simulink model "Demo_Intersection_cs"  (Simulink 7.6)
settings: Solver=FixedStepDiscrete  SolverMode=SingleTasking  StartTime=0.0  StopTime=13  FixedStep=1/20  RelTol=1e-3
PreLoadFcn:
  | check_NUTS_defined
  | model_closed = 0;
  | assignin('base',['model_closed_' bdroot],false);
InitFcn:
  | PreScanExperimentInitFcn(bdroot)
StopFcn:
  | PreScanExperimentStopFcn(bdroot);
  | 
undefined symbols (not defined in the file or in its folder): DiscIntNeverNeededParam
libraries: PreScanSimulinkLibrary x32, PreScanUsefulBlocks x8, simulink_extras x3
(part 5 of 5)

== system Demo_Intersection_cs/Nissan_Cabstar_1/Trajectories/Traj2State3/Traj2State2/Traj2MuxState_Ext ==
  Traj : Inport
  Terminator{1..9} (9 alike) : Terminator
  demux : Subsystem
  x [m] : Outport
  y [m] : Outport  Port=2
  z [m] : Outport  Port=3
  dx [m/s] : Outport  Port=4
  dy [m/s] : Outport  Port=5
  dz [m/s] : Outport  Port=6
  R [rad] : Outport  Port=7
  P [rad] : Outport  Port=8
  Y [rad] : Outport  Port=9
  wires:
  demux/9(Y) -> Y [rad]/1
  demux/7(R) -> R [rad]/1
  demux/5(vely) -> dy [m/s]/1
  demux/4(velx) -> dx [m/s]/1
  demux/10(velR) -> Terminator4/1
  demux/11(velP) -> Terminator5/1
  demux/12(velY) -> Terminator1/1
  demux/13(accx) -> Terminator8/1
  demux/14(accy) -> Terminator9/1
  demux/15(accz) -> Terminator7/1
  demux/18(accY) -> Terminator2/1
  demux/16(accR) -> Terminator3/1
  demux/17(accP) -> Terminator6/1
  demux/3(z) -> z [m]/1
  Traj/1 -> demux/1(traj)
  demux/6(velz) -> dz [m/s]/1
  demux/1(x) -> x [m]/1
  demux/2(y) -> y [m]/1
  demux/8(P) -> P [rad]/1

== system Demo_Intersection_cs/Toyota_Previa_1/Trajectories/Traj2State1/Traj2State2/MuxState ==
  x [m] : Inport
  y [m] : Inport  Port=2
  z [m] : Inport  Port=3
  dx [m/s] : Inport  Port=4
  dy [m/s] : Inport  Port=5
  dz [m/s] : Inport  Port=6
  R [rad] : Inport  Port=7
  P [rad] : Inport  Port=8
  Y [rad] : Inport  Port=9
  Mux : Mux  Inputs=9
  state : Outport
  wires:
  z [m]/1 -> Mux/3
  y [m]/1 -> Mux/2
  x [m]/1 -> Mux/1
  Y [rad]/1 -> Mux/9
  P [rad]/1 -> Mux/8
  R [rad]/1 -> Mux/7
  dz [m/s]/1 -> Mux/6
  dy [m/s]/1 -> Mux/5
  dx [m/s]/1 -> Mux/4
  Mux/1 -> state/1

== system Demo_Intersection_cs/Toyota_Previa_1/Trajectories/Traj2State1/Traj2State2/Traj2MuxState_Ext ==
  Traj : Inport
  Terminator{1..9} (9 alike) : Terminator
  demux : Subsystem
  x [m] : Outport
  y [m] : Outport  Port=2
  z [m] : Outport  Port=3
  dx [m/s] : Outport  Port=4
  dy [m/s] : Outport  Port=5
  dz [m/s] : Outport  Port=6
  R [rad] : Outport  Port=7
  P [rad] : Outport  Port=8
  Y [rad] : Outport  Port=9
  wires:
  demux/9(Y) -> Y [rad]/1
  demux/7(R) -> R [rad]/1
  demux/5(vely) -> dy [m/s]/1
  demux/4(velx) -> dx [m/s]/1
  demux/10(velR) -> Terminator4/1
  demux/11(velP) -> Terminator5/1
  demux/12(velY) -> Terminator1/1
  demux/13(accx) -> Terminator8/1
  demux/14(accy) -> Terminator9/1
  demux/15(accz) -> Terminator7/1
  demux/18(accY) -> Terminator2/1
  demux/16(accR) -> Terminator3/1
  demux/17(accP) -> Terminator6/1
  demux/3(z) -> z [m]/1
  Traj/1 -> demux/1(traj)
  demux/6(velz) -> dz [m/s]/1
  demux/1(x) -> x [m]/1
  demux/2(y) -> y [m]/1
  demux/8(P) -> P [rad]/1

== system Demo_Intersection_cs/Toyota_Previa_1/Trajectories/Traj2State2/Traj2State2/MuxState ==
  x [m] : Inport
  y [m] : Inport  Port=2
  z [m] : Inport  Port=3
  dx [m/s] : Inport  Port=4
  dy [m/s] : Inport  Port=5
  dz [m/s] : Inport  Port=6
  R [rad] : Inport  Port=7
  P [rad] : Inport  Port=8
  Y [rad] : Inport  Port=9
  Mux : Mux  Inputs=9
  state : Outport
  wires:
  z [m]/1 -> Mux/3
  y [m]/1 -> Mux/2
  x [m]/1 -> Mux/1
  Y [rad]/1 -> Mux/9
  P [rad]/1 -> Mux/8
  R [rad]/1 -> Mux/7
  dz [m/s]/1 -> Mux/6
  dy [m/s]/1 -> Mux/5
  dx [m/s]/1 -> Mux/4
  Mux/1 -> state/1

== system Demo_Intersection_cs/Toyota_Previa_1/Trajectories/Traj2State2/Traj2State2/Traj2MuxState_Ext ==
  Traj : Inport
  Terminator{1..9} (9 alike) : Terminator
  demux : Subsystem
  x [m] : Outport
  y [m] : Outport  Port=2
  z [m] : Outport  Port=3
  dx [m/s] : Outport  Port=4
  dy [m/s] : Outport  Port=5
  dz [m/s] : Outport  Port=6
  R [rad] : Outport  Port=7
  P [rad] : Outport  Port=8
  Y [rad] : Outport  Port=9
  wires:
  demux/9(Y) -> Y [rad]/1
  demux/7(R) -> R [rad]/1
  demux/5(vely) -> dy [m/s]/1
  demux/4(velx) -> dx [m/s]/1
  demux/10(velR) -> Terminator4/1
  demux/11(velP) -> Terminator5/1
  demux/12(velY) -> Terminator1/1
  demux/13(accx) -> Terminator8/1
  demux/14(accy) -> Terminator9/1
  demux/15(accz) -> Terminator7/1
  demux/18(accY) -> Terminator2/1
  demux/16(accR) -> Terminator3/1
  demux/17(accP) -> Terminator6/1
  demux/3(z) -> z [m]/1
  Traj/1 -> demux/1(traj)
  demux/6(velz) -> dz [m/s]/1
  demux/1(x) -> x [m]/1
  demux/2(y) -> y [m]/1
  demux/8(P) -> P [rad]/1

== system Demo_Intersection_cs/Toyota_Previa_1/Trajectories/Traj2State3/Traj2State2/MuxState ==
  x [m] : Inport
  y [m] : Inport  Port=2
  z [m] : Inport  Port=3
  dx [m/s] : Inport  Port=4
  dy [m/s] : Inport  Port=5
  dz [m/s] : Inport  Port=6
  R [rad] : Inport  Port=7
  P [rad] : Inport  Port=8
  Y [rad] : Inport  Port=9
  Mux : Mux  Inputs=9
  state : Outport
  wires:
  z [m]/1 -> Mux/3
  y [m]/1 -> Mux/2
  x [m]/1 -> Mux/1
  Y [rad]/1 -> Mux/9
  P [rad]/1 -> Mux/8
  R [rad]/1 -> Mux/7
  dz [m/s]/1 -> Mux/6
  dy [m/s]/1 -> Mux/5
  dx [m/s]/1 -> Mux/4
  Mux/1 -> state/1

== system Demo_Intersection_cs/Toyota_Previa_1/Trajectories/Traj2State3/Traj2State2/Traj2MuxState_Ext ==
  Traj : Inport
  Terminator{1..9} (9 alike) : Terminator
  demux : Subsystem
  x [m] : Outport
  y [m] : Outport  Port=2
  z [m] : Outport  Port=3
  dx [m/s] : Outport  Port=4
  dy [m/s] : Outport  Port=5
  dz [m/s] : Outport  Port=6
  R [rad] : Outport  Port=7
  P [rad] : Outport  Port=8
  Y [rad] : Outport  Port=9
  wires:
  demux/9(Y) -> Y [rad]/1
  demux/7(R) -> R [rad]/1
  demux/5(vely) -> dy [m/s]/1
  demux/4(velx) -> dx [m/s]/1
  demux/10(velR) -> Terminator4/1
  demux/11(velP) -> Terminator5/1
  demux/12(velY) -> Terminator1/1
  demux/13(accx) -> Terminator8/1
  demux/14(accy) -> Terminator9/1
  demux/15(accz) -> Terminator7/1
  demux/18(accY) -> Terminator2/1
  demux/16(accR) -> Terminator3/1
  demux/17(accP) -> Terminator6/1
  demux/3(z) -> z [m]/1
  Traj/1 -> demux/1(traj)
  demux/6(velz) -> dz [m/s]/1
  demux/1(x) -> x [m]/1
  demux/2(y) -> y [m]/1
  demux/8(P) -> P [rad]/1

== system Demo_Intersection_cs/Toyota_Yaris_1/Trajectories/Traj2State1/Traj2State2/MuxState ==
  x [m] : Inport
  y [m] : Inport  Port=2
  z [m] : Inport  Port=3
  dx [m/s] : Inport  Port=4
  dy [m/s] : Inport  Port=5
  dz [m/s] : Inport  Port=6
  R [rad] : Inport  Port=7
  P [rad] : Inport  Port=8
  Y [rad] : Inport  Port=9
  Mux : Mux  Inputs=9
  state : Outport
  wires:
  z [m]/1 -> Mux/3
  y [m]/1 -> Mux/2
  x [m]/1 -> Mux/1
  Y [rad]/1 -> Mux/9
  P [rad]/1 -> Mux/8
  R [rad]/1 -> Mux/7
  dz [m/s]/1 -> Mux/6
  dy [m/s]/1 -> Mux/5
  dx [m/s]/1 -> Mux/4
  Mux/1 -> state/1

== system Demo_Intersection_cs/Toyota_Yaris_1/Trajectories/Traj2State1/Traj2State2/Traj2MuxState_Ext ==
  Traj : Inport
  Terminator{1..9} (9 alike) : Terminator
  demux : Subsystem
  x [m] : Outport
  y [m] : Outport  Port=2
  z [m] : Outport  Port=3
  dx [m/s] : Outport  Port=4
  dy [m/s] : Outport  Port=5
  dz [m/s] : Outport  Port=6
  R [rad] : Outport  Port=7
  P [rad] : Outport  Port=8
  Y [rad] : Outport  Port=9
  wires:
  demux/9(Y) -> Y [rad]/1
  demux/7(R) -> R [rad]/1
  demux/5(vely) -> dy [m/s]/1
  demux/4(velx) -> dx [m/s]/1
  demux/10(velR) -> Terminator4/1
  demux/11(velP) -> Terminator5/1
  demux/12(velY) -> Terminator1/1
  demux/13(accx) -> Terminator8/1
  demux/14(accy) -> Terminator9/1
  demux/15(accz) -> Terminator7/1
  demux/18(accY) -> Terminator2/1
  demux/16(accR) -> Terminator3/1
  demux/17(accP) -> Terminator6/1
  demux/3(z) -> z [m]/1
  Traj/1 -> demux/1(traj)
  demux/6(velz) -> dz [m/s]/1
  demux/1(x) -> x [m]/1
  demux/2(y) -> y [m]/1
  demux/8(P) -> P [rad]/1

== system Demo_Intersection_cs/Toyota_Yaris_1/Trajectories/Traj2State2/Traj2State2/MuxState ==
  x [m] : Inport
  y [m] : Inport  Port=2
  z [m] : Inport  Port=3
  dx [m/s] : Inport  Port=4
  dy [m/s] : Inport  Port=5
  dz [m/s] : Inport  Port=6
  R [rad] : Inport  Port=7
  P [rad] : Inport  Port=8
  Y [rad] : Inport  Port=9
  Mux : Mux  Inputs=9
  state : Outport
  wires:
  z [m]/1 -> Mux/3
  y [m]/1 -> Mux/2
  x [m]/1 -> Mux/1
  Y [rad]/1 -> Mux/9
  P [rad]/1 -> Mux/8
  R [rad]/1 -> Mux/7
  dz [m/s]/1 -> Mux/6
  dy [m/s]/1 -> Mux/5
  dx [m/s]/1 -> Mux/4
  Mux/1 -> state/1

== system Demo_Intersection_cs/Toyota_Yaris_1/Trajectories/Traj2State2/Traj2State2/Traj2MuxState_Ext ==
  Traj : Inport
  Terminator{1..9} (9 alike) : Terminator
  demux : Subsystem
  x [m] : Outport
  y [m] : Outport  Port=2
  z [m] : Outport  Port=3
  dx [m/s] : Outport  Port=4
  dy [m/s] : Outport  Port=5
  dz [m/s] : Outport  Port=6
  R [rad] : Outport  Port=7
  P [rad] : Outport  Port=8
  Y [rad] : Outport  Port=9
  wires:
  demux/9(Y) -> Y [rad]/1
  demux/7(R) -> R [rad]/1
  demux/5(vely) -> dy [m/s]/1
  demux/4(velx) -> dx [m/s]/1
  demux/10(velR) -> Terminator4/1
  demux/11(velP) -> Terminator5/1
  demux/12(velY) -> Terminator1/1
  demux/13(accx) -> Terminator8/1
  demux/14(accy) -> Terminator9/1
  demux/15(accz) -> Terminator7/1
  demux/18(accY) -> Terminator2/1
  demux/16(accR) -> Terminator3/1
  demux/17(accP) -> Terminator6/1
  demux/3(z) -> z [m]/1
  Traj/1 -> demux/1(traj)
  demux/6(velz) -> dz [m/s]/1
  demux/1(x) -> x [m]/1
  demux/2(y) -> y [m]/1
  demux/8(P) -> P [rad]/1

== system Demo_Intersection_cs/Toyota_Yaris_1/Trajectories/Traj2State3/Traj2State2/MuxState ==
  x [m] : Inport
  y [m] : Inport  Port=2
  z [m] : Inport  Port=3
  dx [m/s] : Inport  Port=4
  dy [m/s] : Inport  Port=5
  dz [m/s] : Inport  Port=6
  R [rad] : Inport  Port=7
  P [rad] : Inport  Port=8
  Y [rad] : Inport  Port=9
  Mux : Mux  Inputs=9
  state : Outport
  wires:
  z [m]/1 -> Mux/3
  y [m]/1 -> Mux/2
  x [m]/1 -> Mux/1
  Y [rad]/1 -> Mux/9
  P [rad]/1 -> Mux/8
  R [rad]/1 -> Mux/7
  dz [m/s]/1 -> Mux/6
  dy [m/s]/1 -> Mux/5
  dx [m/s]/1 -> Mux/4
  Mux/1 -> state/1

== system Demo_Intersection_cs/Toyota_Yaris_1/Trajectories/Traj2State3/Traj2State2/Traj2MuxState_Ext ==
  Traj : Inport
  Terminator{1..9} (9 alike) : Terminator
  demux : Subsystem
  x [m] : Outport
  y [m] : Outport  Port=2
  z [m] : Outport  Port=3
  dx [m/s] : Outport  Port=4
  dy [m/s] : Outport  Port=5
  dz [m/s] : Outport  Port=6
  R [rad] : Outport  Port=7
  P [rad] : Outport  Port=8
  Y [rad] : Outport  Port=9
  wires:
  demux/9(Y) -> Y [rad]/1
  demux/7(R) -> R [rad]/1
  demux/5(vely) -> dy [m/s]/1
  demux/4(velx) -> dx [m/s]/1
  demux/10(velR) -> Terminator4/1
  demux/11(velP) -> Terminator5/1
  demux/12(velY) -> Terminator1/1
  demux/13(accx) -> Terminator8/1
  demux/14(accy) -> Terminator9/1
  demux/15(accz) -> Terminator7/1
  demux/18(accY) -> Terminator2/1
  demux/16(accR) -> Terminator3/1
  demux/17(accP) -> Terminator6/1
  demux/3(z) -> z [m]/1
  Traj/1 -> demux/1(traj)
  demux/6(velz) -> dz [m/s]/1
  demux/1(x) -> x [m]/1
  demux/2(y) -> y [m]/1
  demux/8(P) -> P [rad]/1

== system Demo_Intersection_cs/Nissan_Cabstar_1/Trajectories/Traj2State1/Traj2State2/Traj2MuxState_Ext/demux ==
  traj : Inport
  Demux : Demux  Outputs=18
  x : Outport
  y : Outport  Port=2
  z : Outport  Port=3
  velx : Outport  Port=4
  vely : Outport  Port=5
  velz : Outport  Port=6
  R : Outport  Port=7
  P : Outport  Port=8
  Y : Outport  Port=9
  velR : Outport  Port=10
  velP : Outport  Port=11
  velY : Outport  Port=12
  accx : Outport  Port=13
  accy : Outport  Port=14
  accz : Outport  Port=15
  accR : Outport  Port=16
  accP : Outport  Port=17
  accY : Outport  Port=18
  wires:
  Demux/18 -> accY/1
  Demux/17 -> accP/1
  Demux/16 -> accR/1
  Demux/15 -> accz/1
  Demux/14 -> accy/1
  Demux/13 -> accx/1
  Demux/12 -> velY/1
  Demux/11 -> velP/1
  Demux/10 -> velR/1
  Demux/9 -> velz/1
  Demux/8 -> vely/1
  Demux/7 -> velx/1
  Demux/6 -> Y/1
  Demux/5 -> P/1
  traj/1 -> Demux/1
  Demux/4 -> R/1
  Demux/3 -> z/1
  Demux/2 -> y/1
  Demux/1 -> x/1

== system Demo_Intersection_cs/Nissan_Cabstar_1/Trajectories/Traj2State2/Traj2State2/Traj2MuxState_Ext/demux ==
  traj : Inport
  Demux : Demux  Outputs=18
  x : Outport
  y : Outport  Port=2
  z : Outport  Port=3
  velx : Outport  Port=4
  vely : Outport  Port=5
  velz : Outport  Port=6
  R : Outport  Port=7
  P : Outport  Port=8
  Y : Outport  Port=9
  velR : Outport  Port=10
  velP : Outport  Port=11
  velY : Outport  Port=12
  accx : Outport  Port=13
  accy : Outport  Port=14
  accz : Outport  Port=15
  accR : Outport  Port=16
  accP : Outport  Port=17
  accY : Outport  Port=18
  wires:
  Demux/18 -> accY/1
  Demux/17 -> accP/1
  Demux/16 -> accR/1
  Demux/15 -> accz/1
  Demux/14 -> accy/1
  Demux/13 -> accx/1
  Demux/12 -> velY/1
  Demux/11 -> velP/1
  Demux/10 -> velR/1
  Demux/9 -> velz/1
  Demux/8 -> vely/1
  Demux/7 -> velx/1
  Demux/6 -> Y/1
  Demux/5 -> P/1
  traj/1 -> Demux/1
  Demux/4 -> R/1
  Demux/3 -> z/1
  Demux/2 -> y/1
  Demux/1 -> x/1

== system Demo_Intersection_cs/Nissan_Cabstar_1/Trajectories/Traj2State3/Traj2State2/Traj2MuxState_Ext/demux ==
  traj : Inport
  Demux : Demux  Outputs=18
  x : Outport
  y : Outport  Port=2
  z : Outport  Port=3
  velx : Outport  Port=4
  vely : Outport  Port=5
  velz : Outport  Port=6
  R : Outport  Port=7
  P : Outport  Port=8
  Y : Outport  Port=9
  velR : Outport  Port=10
  velP : Outport  Port=11
  velY : Outport  Port=12
  accx : Outport  Port=13
  accy : Outport  Port=14
  accz : Outport  Port=15
  accR : Outport  Port=16
  accP : Outport  Port=17
  accY : Outport  Port=18
  wires:
  Demux/18 -> accY/1
  Demux/17 -> accP/1
  Demux/16 -> accR/1
  Demux/15 -> accz/1
  Demux/14 -> accy/1
  Demux/13 -> accx/1
  Demux/12 -> velY/1
  Demux/11 -> velP/1
  Demux/10 -> velR/1
  Demux/9 -> velz/1
  Demux/8 -> vely/1
  Demux/7 -> velx/1
  Demux/6 -> Y/1
  Demux/5 -> P/1
  traj/1 -> Demux/1
  Demux/4 -> R/1
  Demux/3 -> z/1
  Demux/2 -> y/1
  Demux/1 -> x/1

== system Demo_Intersection_cs/Toyota_Previa_1/Trajectories/Traj2State1/Traj2State2/Traj2MuxState_Ext/demux ==
  traj : Inport
  Demux : Demux  Outputs=18
  x : Outport
  y : Outport  Port=2
  z : Outport  Port=3
  velx : Outport  Port=4
  vely : Outport  Port=5
  velz : Outport  Port=6
  R : Outport  Port=7
  P : Outport  Port=8
  Y : Outport  Port=9
  velR : Outport  Port=10
  velP : Outport  Port=11
  velY : Outport  Port=12
  accx : Outport  Port=13
  accy : Outport  Port=14
  accz : Outport  Port=15
  accR : Outport  Port=16
  accP : Outport  Port=17
  accY : Outport  Port=18
  wires:
  Demux/18 -> accY/1
  Demux/17 -> accP/1
  Demux/16 -> accR/1
  Demux/15 -> accz/1
  Demux/14 -> accy/1
  Demux/13 -> accx/1
  Demux/12 -> velY/1
  Demux/11 -> velP/1
  Demux/10 -> velR/1
  Demux/9 -> velz/1
  Demux/8 -> vely/1
  Demux/7 -> velx/1
  Demux/6 -> Y/1
  Demux/5 -> P/1
  traj/1 -> Demux/1
  Demux/4 -> R/1
  Demux/3 -> z/1
  Demux/2 -> y/1
  Demux/1 -> x/1

== system Demo_Intersection_cs/Toyota_Previa_1/Trajectories/Traj2State2/Traj2State2/Traj2MuxState_Ext/demux ==
  traj : Inport
  Demux : Demux  Outputs=18
  x : Outport
  y : Outport  Port=2
  z : Outport  Port=3
  velx : Outport  Port=4
  vely : Outport  Port=5
  velz : Outport  Port=6
  R : Outport  Port=7
  P : Outport  Port=8
  Y : Outport  Port=9
  velR : Outport  Port=10
  velP : Outport  Port=11
  velY : Outport  Port=12
  accx : Outport  Port=13
  accy : Outport  Port=14
  accz : Outport  Port=15
  accR : Outport  Port=16
  accP : Outport  Port=17
  accY : Outport  Port=18
  wires:
  Demux/18 -> accY/1
  Demux/17 -> accP/1
  Demux/16 -> accR/1
  Demux/15 -> accz/1
  Demux/14 -> accy/1
  Demux/13 -> accx/1
  Demux/12 -> velY/1
  Demux/11 -> velP/1
  Demux/10 -> velR/1
  Demux/9 -> velz/1
  Demux/8 -> vely/1
  Demux/7 -> velx/1
  Demux/6 -> Y/1
  Demux/5 -> P/1
  traj/1 -> Demux/1
  Demux/4 -> R/1
  Demux/3 -> z/1
  Demux/2 -> y/1
  Demux/1 -> x/1

== system Demo_Intersection_cs/Toyota_Previa_1/Trajectories/Traj2State3/Traj2State2/Traj2MuxState_Ext/demux ==
  traj : Inport
  Demux : Demux  Outputs=18
  x : Outport
  y : Outport  Port=2
  z : Outport  Port=3
  velx : Outport  Port=4
  vely : Outport  Port=5
  velz : Outport  Port=6
  R : Outport  Port=7
  P : Outport  Port=8
  Y : Outport  Port=9
  velR : Outport  Port=10
  velP : Outport  Port=11
  velY : Outport  Port=12
  accx : Outport  Port=13
  accy : Outport  Port=14
  accz : Outport  Port=15
  accR : Outport  Port=16
  accP : Outport  Port=17
  accY : Outport  Port=18
  wires:
  Demux/18 -> accY/1
  Demux/17 -> accP/1
  Demux/16 -> accR/1
  Demux/15 -> accz/1
  Demux/14 -> accy/1
  Demux/13 -> accx/1
  Demux/12 -> velY/1
  Demux/11 -> velP/1
  Demux/10 -> velR/1
  Demux/9 -> velz/1
  Demux/8 -> vely/1
  Demux/7 -> velx/1
  Demux/6 -> Y/1
  Demux/5 -> P/1
  traj/1 -> Demux/1
  Demux/4 -> R/1
  Demux/3 -> z/1
  Demux/2 -> y/1
  Demux/1 -> x/1

== system Demo_Intersection_cs/Toyota_Yaris_1/Trajectories/Traj2State1/Traj2State2/Traj2MuxState_Ext/demux ==
  traj : Inport
  Demux : Demux  Outputs=18
  x : Outport
  y : Outport  Port=2
  z : Outport  Port=3
  velx : Outport  Port=4
  vely : Outport  Port=5
  velz : Outport  Port=6
  R : Outport  Port=7
  P : Outport  Port=8
  Y : Outport  Port=9
  velR : Outport  Port=10
  velP : Outport  Port=11
  velY : Outport  Port=12
  accx : Outport  Port=13
  accy : Outport  Port=14
  accz : Outport  Port=15
  accR : Outport  Port=16
  accP : Outport  Port=17
  accY : Outport  Port=18
  wires:
  Demux/18 -> accY/1
  Demux/17 -> accP/1
  Demux/16 -> accR/1
  Demux/15 -> accz/1
  Demux/14 -> accy/1
  Demux/13 -> accx/1
  Demux/12 -> velY/1
  Demux/11 -> velP/1
  Demux/10 -> velR/1
  Demux/9 -> velz/1
  Demux/8 -> vely/1
  Demux/7 -> velx/1
  Demux/6 -> Y/1
  Demux/5 -> P/1
  traj/1 -> Demux/1
  Demux/4 -> R/1
  Demux/3 -> z/1
  Demux/2 -> y/1
  Demux/1 -> x/1

== system Demo_Intersection_cs/Toyota_Yaris_1/Trajectories/Traj2State2/Traj2State2/Traj2MuxState_Ext/demux ==
  traj : Inport
  Demux : Demux  Outputs=18
  x : Outport
  y : Outport  Port=2
  z : Outport  Port=3
  velx : Outport  Port=4
  vely : Outport  Port=5
  velz : Outport  Port=6
  R : Outport  Port=7
  P : Outport  Port=8
  Y : Outport  Port=9
  velR : Outport  Port=10
  velP : Outport  Port=11
  velY : Outport  Port=12
  accx : Outport  Port=13
  accy : Outport  Port=14
  accz : Outport  Port=15
  accR : Outport  Port=16
  accP : Outport  Port=17
  accY : Outport  Port=18
  wires:
  Demux/18 -> accY/1
  Demux/17 -> accP/1
  Demux/16 -> accR/1
  Demux/15 -> accz/1
  Demux/14 -> accy/1
  Demux/13 -> accx/1
  Demux/12 -> velY/1
  Demux/11 -> velP/1
  Demux/10 -> velR/1
  Demux/9 -> velz/1
  Demux/8 -> vely/1
  Demux/7 -> velx/1
  Demux/6 -> Y/1
  Demux/5 -> P/1
  traj/1 -> Demux/1
  Demux/4 -> R/1
  Demux/3 -> z/1
  Demux/2 -> y/1
  Demux/1 -> x/1

== system Demo_Intersection_cs/Toyota_Yaris_1/Trajectories/Traj2State3/Traj2State2/Traj2MuxState_Ext/demux ==
  traj : Inport
  Demux : Demux  Outputs=18
  x : Outport
  y : Outport  Port=2
  z : Outport  Port=3
  velx : Outport  Port=4
  vely : Outport  Port=5
  velz : Outport  Port=6
  R : Outport  Port=7
  P : Outport  Port=8
  Y : Outport  Port=9
  velR : Outport  Port=10
  velP : Outport  Port=11
  velY : Outport  Port=12
  accx : Outport  Port=13
  accy : Outport  Port=14
  accz : Outport  Port=15
  accR : Outport  Port=16
  accP : Outport  Port=17
  accY : Outport  Port=18
  wires:
  Demux/18 -> accY/1
  Demux/17 -> accP/1
  Demux/16 -> accR/1
  Demux/15 -> accz/1
  Demux/14 -> accy/1
  Demux/13 -> accx/1
  Demux/12 -> velY/1
  Demux/11 -> velP/1
  Demux/10 -> velR/1
  Demux/9 -> velz/1
  Demux/8 -> vely/1
  Demux/7 -> velx/1
  Demux/6 -> Y/1
  Demux/5 -> P/1
  traj/1 -> Demux/1
  Demux/4 -> R/1
  Demux/3 -> z/1
  Demux/2 -> y/1
  Demux/1 -> x/1

== matlab function Mazda_RX8_1/Sort AIR Output based on ID/Embedded MATLAB Function ==
  data: u input double; y output double; mode input double; ignorezero input double; ids input double
function y = fcn(u,mode, ignorezero, ids)
% This block supports an embeddable subset of the MATLAB language.
% See the help menu for details. 

[a,y] = sort(u);
if mode == 2 %'descend'
    y=y(end:-1:1);
end

if mode == 1 && ignorezero == 1 
    ly = length(y);
    % ignore zero detections (NB: not required for descending)
    % => place zero detections at end
% TODO: preferred implementation: not available yet in 2006a
%     A=logical(ids(y)~=0);
%     y=[y(A); y(~A)]';
    index=ly+1;
    base=0; %temp value to fix issue with loop variable i
    indices = zeros(1,ly);
    for i=1:ly
        base=i;
        if ids(y(i)) ~= 0
            index = i;
            break
        end
    end
    for i=1:ly-index+1
        indices(i) = index+i-1;
    end
    if index==ly+1;
        base=0;
    end
    for j=1:index-1
        indices(base+j)=j;
    end
    y=y(indices);
end

== stateflow chart Mazda_RX8_1/Decision Algorithm ==
  state Decision_algorithm
    state CAR1 [parallel]
      settings: executionOrder=2
      state Lane1
        state RightTurn
          en: W[1]=WM[1];
        state Straight
          en: W[1]=WM[2];
        state LeftTurn
          en: W[1]=WM[3];
        (default) -> (junction 56) [order 1]
        (junction 56) -> Decision_algorithm.CAR1.Lane1.Straight [order 2] : [C1[3]==0]
        (junction 56) -> Decision_algorithm.CAR1.Lane1.LeftTurn [order 1] : [C1[3]<0]
        (junction 56) -> Decision_algorithm.CAR1.Lane1.RightTurn [order 3] : [C1[3]>0]
        (default) -> Decision_algorithm.CAR1.Lane1.Straight [order 2]
      state Lane2
        state LeftTurn
          en: W[2]=WM[6];
        state Straight
          en: W[2]=WM[5];
        state RightTurn
          en: W[2]=WM[4];
        (default) -> (junction 57) [order 1]
        (junction 57) -> Decision_algorithm.CAR1.Lane2.RightTurn [order 3] : [C1[3]>0]
        (junction 57) -> Decision_algorithm.CAR1.Lane2.LeftTurn [order 1] : [C1[3]<0]
        (junction 57) -> Decision_algorithm.CAR1.Lane2.Straight [order 2] : [C1[3]==0]
        (default) -> Decision_algorithm.CAR1.Lane2.Straight [order 2]
      state Enter
      state Lane3
        state RightTurn
          en: W[3]=WM[7];
        state Straight
          en: W[3]=WM[8];
        state LeftTurn
          en: W[3]=WM[9];
        (junction 58) -> Decision_algorithm.CAR1.Lane3.RightTurn [order 1] : [C1[3]>0]
        (junction 58) -> Decision_algorithm.CAR1.Lane3.Straight [order 3] : [C1[3]==0]
        (junction 58) -> Decision_algorithm.CAR1.Lane3.LeftTurn [order 2] : [C1[3]<0]
        (default) -> (junction 58) [order 1]
        (default) -> Decision_algorithm.CAR1.Lane3.Straight [order 2]
      Decision_algorithm.CAR1.Enter -> Decision_algorithm.CAR1.Lane3 [order 2] : [C1[2]>-135 && C1[2]<-90 && C1[1]<Rcross...
          | && ((C1[4]>315 && C1[4]<=360) ||...
          | (C1[4]>=0 && C1[4]<45))]
      Decision_algorithm.CAR1.Enter -> Decision_algorithm.CAR1.Lane1 [order 3] : [C1[2]>45 && C1[2]<90 && C1[1]<Rcross...
          | && C1[4]>135 && C1[4]<225]
      Decision_algorithm.CAR1.Enter -> Decision_algorithm.CAR1.Lane2 [order 1] : [C1[2]>-45 && C1[2]<0 && C1[1]<Rcross...
          | && C1[4]>225 && C1[4]<315]
      (default) -> Decision_algorithm.CAR1.Enter : {W[1]=0;
          | W[2]=0;
          | W[3]=0;}
      Decision_algorithm.CAR1.Lane3.Straight -> Decision_algorithm.CAR1.Enter
      Decision_algorithm.CAR1.Lane3.RightTurn -> Decision_algorithm.CAR1.Enter
      Decision_algorithm.CAR1.Lane2.RightTurn -> Decision_algorithm.CAR1.Enter
      Decision_algorithm.CAR1.Lane1.RightTurn -> Decision_algorithm.CAR1.Enter
      Decision_algorithm.CAR1.Lane2.LeftTurn -> Decision_algorithm.CAR1.Enter
      Decision_algorithm.CAR1.Lane2.Straight -> Decision_algorithm.CAR1.Enter
      Decision_algorithm.CAR1.Lane1.Straight -> Decision_algorithm.CAR1.Enter
      Decision_algorithm.CAR1.Lane1.LeftTurn -> Decision_algorithm.CAR1.Enter
      Decision_algorithm.CAR1.Lane3.LeftTurn -> Decision_algorithm.CAR1.Enter
      Decision_algorithm.CAR1.Enter -> Decision_algorithm.CAR1.Enter [order 4] : {W[1]=0;
          | W[2]=0;
          | W[3]=0;}
    state CAR2 [parallel]
      settings: executionOrder=1
      state Lane2
        state LeftTurn
          en: W[5]=WM[6];
        state Straight
          en: W[5]=WM[5];
        state RightTurn
          en: W[5]=WM[4];
        (junction 60) -> Decision_algorithm.CAR2.Lane2.Straight [order 2] : [C2[3]==0]
        (junction 60) -> Decision_algorithm.CAR2.Lane2.LeftTurn [order 1] : [C2[3]<0]
        (junction 60) -> Decision_algorithm.CAR2.Lane2.RightTurn [order 3] : [C2[3]>0]
        (default) -> (junction 60) [order 1]
        (default) -> Decision_algorithm.CAR2.Lane2.Straight [order 2]
      state Lane1
        state RightTurn
          en: W[4]=WM[1];
        state Straight
          en: W[4]=WM[2];
        state LeftTurn
          en: W[4]=WM[3];
        (junction 61) -> Decision_algorithm.CAR2.Lane1.RightTurn [order 2] : [C2[3]>0]
        (junction 61) -> Decision_algorithm.CAR2.Lane1.LeftTurn [order 3] : [C2[3]<0]
        (junction 61) -> Decision_algorithm.CAR2.Lane1.Straight [order 1] : [C2[3]==0]
        (default) -> (junction 61) [order 1]
        (default) -> Decision_algorithm.CAR2.Lane1.Straight [order 2]
      state Lane3
        state LeftTurn
          en: W[6]=WM[9];
        state Straight
          en: W[6]=WM[8];
        state RightTurn
          en: W[6]=WM[7];
        (default) -> (junction 59) [order 1]
        (junction 59) -> Decision_algorithm.CAR2.Lane3.LeftTurn [order 2] : [C2[3]<0]
        (junction 59) -> Decision_algorithm.CAR2.Lane3.Straight [order 3] : [C2[3]==0]
        (junction 59) -> Decision_algorithm.CAR2.Lane3.RightTurn [order 1] : [C2[3]>0]
        (default) -> Decision_algorithm.CAR2.Lane3.Straight [order 2]
      state Enter
      Decision_algorithm.CAR2.Lane3.Straight -> Decision_algorithm.CAR2.Enter
      (default) -> Decision_algorithm.CAR2.Enter : {W[4]=0;
          | W[5]=0;
          | W[6]=0;}
      Decision_algorithm.CAR2.Enter -> Decision_algorithm.CAR2.Lane2 [order 1] : [C2[2]>-45 && C2[2]<0 && C2[1]<Rcross...
          | && C2[4]>225 && C2[4]<315]
      Decision_algorithm.CAR2.Enter -> Decision_algorithm.CAR2.Lane1 [order 3] : [C2[2]>45 && C2[2]<90 && C2[1]<Rcross...
          | && C2[4]>135 && C2[4]<225]
      Decision_algorithm.CAR2.Enter -> Decision_algorithm.CAR2.Lane3 [order 2] : [C2[2]>-135 && C2[2]<-90 && C2[1]<Rcross...
          | && ((C2[4]>315 && C2[4]<=360) ||...
          | (C2[4]>=0 && C2[4]<45))]
      Decision_algorithm.CAR2.Lane2.RightTurn -> Decision_algorithm.CAR2.Enter
      Decision_algorithm.CAR2.Lane1.RightTurn -> Decision_algorithm.CAR2.Enter
      Decision_algorithm.CAR2.Lane3.RightTurn -> Decision_algorithm.CAR2.Enter
      Decision_algorithm.CAR2.Lane3.LeftTurn -> Decision_algorithm.CAR2.Enter
      Decision_algorithm.CAR2.Lane1.LeftTurn -> Decision_algorithm.CAR2.Enter
      Decision_algorithm.CAR2.Lane1.Straight -> Decision_algorithm.CAR2.Enter
      Decision_algorithm.CAR2.Lane2.Straight -> Decision_algorithm.CAR2.Enter
      Decision_algorithm.CAR2.Lane2.LeftTurn -> Decision_algorithm.CAR2.Enter
      Decision_algorithm.CAR2.Enter -> Decision_algorithm.CAR2.Enter [order 4] : {W[4]=0;
          | W[5]=0;
          | W[6]=0;}
    state CAR3 [parallel]
      settings: executionOrder=3
      state Enter
      state Lane3
        state LeftTurn
          en: W[9]=WM[9];
        state Straight
          en: W[9]=WM[8];
        state RightTurn
          en: W[9]=WM[7];
        (default) -> (junction 63) [order 1]
        (junction 63) -> Decision_algorithm.CAR3.Lane3.Straight [order 3] : [C3[3]==0]
        (junction 63) -> Decision_algorithm.CAR3.Lane3.LeftTurn [order 2] : [C3[3]<0]
        (junction 63) -> Decision_algorithm.CAR3.Lane3.RightTurn [order 1] : [C3[3]>0]
        (default) -> Decision_algorithm.CAR3.Lane3.Straight [order 2]
      state Lane2
        state LeftTurn
          en: W[8]=WM[6];
        state Straight
          en: W[8]=WM[5];
        state RightTurn
          en: W[8]=WM[4];
        (junction 64) -> Decision_algorithm.CAR3.Lane2.RightTurn [order 3] : [C3[3]>0]
        (junction 64) -> Decision_algorithm.CAR3.Lane2.Straight [order 2] : [C3[3]==0]
        (junction 64) -> Decision_algorithm.CAR3.Lane2.LeftTurn [order 1] : [C3[3]<0]
        (default) -> (junction 64) [order 1]
        (default) -> Decision_algorithm.CAR3.Lane2.Straight [order 2]
      state Lane1
        state RightTurn
          en: W[7]=WM[1];
        state LeftTurn
          en: W[7]=WM[3];
        state Straight
          en: W[7]=WM[2];
        (junction 62) -> Decision_algorithm.CAR3.Lane1.LeftTurn [order 3] : [C3[3]<0]
        (junction 62) -> Decision_algorithm.CAR3.Lane1.Straight [order 1] : [C3[3]==0]
        (default) -> (junction 62) [order 1]
        (junction 62) -> Decision_algorithm.CAR3.Lane1.RightTurn [order 2] : [C3[3]>0]
        (default) -> Decision_algorithm.CAR3.Lane1.Straight [order 2]
      Decision_algorithm.CAR3.Lane1.Straight -> Decision_algorithm.CAR3.Enter
      Decision_algorithm.CAR3.Lane3.LeftTurn -> Decision_algorithm.CAR3.Enter
      Decision_algorithm.CAR3.Lane3.Straight -> Decision_algorithm.CAR3.Enter
      Decision_algorithm.CAR3.Lane3.RightTurn -> Decision_algorithm.CAR3.Enter
      Decision_algorithm.CAR3.Lane1.LeftTurn -> Decision_algorithm.CAR3.Enter
      Decision_algorithm.CAR3.Enter -> Decision_algorithm.CAR3.Lane1 [order 3] : [C3[2]>45 && C3[2]<90 && C3[1]<Rcross...
          | && C3[4]>135 && C3[4]<225]
      Decision_algorithm.CAR3.Enter -> Decision_algorithm.CAR3.Lane2 [order 1] : [C3[2]>-45 && C3[2]<0 && C3[1]<Rcross...
          | && C3[4]>225 && C3[4]<315]
      Decision_algorithm.CAR3.Lane2.LeftTurn -> Decision_algorithm.CAR3.Enter
      Decision_algorithm.CAR3.Lane2.Straight -> Decision_algorithm.CAR3.Enter
      Decision_algorithm.CAR3.Lane2.RightTurn -> Decision_algorithm.CAR3.Enter
      Decision_algorithm.CAR3.Enter -> Decision_algorithm.CAR3.Lane3 [order 2] : [C3[2]>-135 && C3[2]<-90 && C3[1]<Rcross...
          | && ((C3[4]>315 && C3[4]<=360) ||...
          | (C3[4]>=0 && C3[4]<45))]
      (default) -> Decision_algorithm.CAR3.Enter : {W[7]=0;
          | W[8]=0;
          | W[9]=0;}
      Decision_algorithm.CAR3.Lane1.RightTurn -> Decision_algorithm.CAR3.Enter
      Decision_algorithm.CAR3.Enter -> Decision_algorithm.CAR3.Enter [order 4] : {W[7]=0;
          | W[8]=0;
          | W[9]=0;}
  data: WM input double size=9; Rcross input double; C1 input double size=4; C2 input double size=4; W output boolean size=9; C3 input double size=4
